simulink model "cm_sat_model"  (R2021b)
settings: Solver=ode23s  StartTime=0.0  StopTime=0.2  FixedStep=0.0001  MaxStep=1e-3  RelTol=5e-7  AbsTol=5e-7  EnableMultiTasking=on
values from neighbouring files (symbols this model uses):
  Dpsi = [ -2454.6 -2412.6 -2370.5 -2328.5 -2286.4 -2244.4 -2202.3  -2160.3 -2118.2 -2076.1 -2034.1 -1992.0 -1950.0 -1907.9 -1865.9  -1823.8 -1781.8 -1739.7 -1697.7 -1655.6 -1613.6 -1571.5 -1529.5  -1487.4 -1445.3 -1403.3 -1361.2 -1319.2 -1277.1 -1235.1 -1193.0  -1151.0 -1108.9 -1066.9 -1024.8 -982.76 -940.71 -898.65 -856.60  -814.55 -772.49 -730.44 -688.39 -646.43 -604.66 -562.89 -521.30  -479.53 -438.14  ...(+559 chars)    [cm_init.m]
  PAR = [wb r1 rp2 xl1 xlp2 xm]    [cm_init.m]
  psisat = [ -170.21 -169.93 -169.65 -169.36 -169.08 -168.80 -168.52  -168.23 -167.95 -167.67 -167.38 -167.10 -166.82 -166.54 -166.25  -165.97 -165.69 -165.40 -165.12 -164.84 -164.56 -164.27 -163.99  -163.71 -163.43 -163.14 -162.86 -162.58 -162.29 -162.01 -161.73  -161.45 -161.16 -160.88 -160.60 -160.32 -160.03 -159.75 -159.47  -159.18 -158.90 -158.62 -158.34 -157.96 -157.39 -156.83 -156.07  -155.51 -154.57  ...(+561 chars)    [cm_init.m]
  wb = 2*pi*F    (= 376.991118431)    [cm_init.m]
  XINIT = [0]    [cm_init.m]
undefined symbols (not defined in the file or in its folder): V1, V1f
settings Model: Creator=Alberto  LastModifiedBy=DELL
settings SolverCC: AutoScaleAbsTol=off  MaxOrder=4  AlgebraicLoopSolver=TrustRegion
settings DataIOCC: LimitDataPoints=on  SaveFormat=Array  SignalLoggingSaveFormat=ModelDataLogs  ReturnWorkspaceOutputs=off  SignalLoggingName=sigsOut
settings OptimizationCC: ExpressionDepthLimit=2147483647  LifeSpan=inf
settings DebuggingCC: AlgebraicLoopMsg=none  SaveWithParameterizedLinksMsg=none  UnderspecifiedInitializationDetection=Classic  MergeDetectMultiDrivingBlocksExec=none  SignalResolutionControl=TryResolveAllWithWarning  MultiTaskDSMMsg=warning  MultiTaskCondExecSysMsg=none  FcnCallInpInsideContextMsg=warning  StateNameClashWarn=warning  SFUnexpectedBacktrackingDiag=warning  SFNoUnconditionalDefaultTransitionDiag=warning  SFExecutionAtInitializationDiag=none  SFMachineParentedDataDiag=warning  ArithmeticOperatorsInVariantConditions=warning
settings HardwareCC: ProdBitPerPointer=32  ProdBitPerSizeT=32  ProdBitPerPtrDiffT=32  ProdLargestAtomicFloat=None  ProdIntDivRoundTo=Undefined  ProdEndianess=Unspecified  ProdWordSize=32  ProdHWDeviceType=32-bit Generic  TargetUnknown=on
settings ModelReferenceCC: PropagateSignalLabelsOutOfModel=off
settings SFSimCC: SimUseLocalCustomCode=off  CustomCodeUndefinedFunction=UseInterfaceOnly
settings RTWCC: RTWUseLocalCustomCode=off
settings CodeAppCC: StateflowObjectComments=on
settings GRTTargetCC: TargetLangStandard=C89/C90 (ANSI)  CombineOutputUpdateFcns=off  GRTInterface=on
settings ConfigComp: CovMetricSettings=dw  CovSaveCumulativeToWorkspaceVar=on  CovSaveSingleToWorkspaceVar=on  CovExternalEMLEnable=off

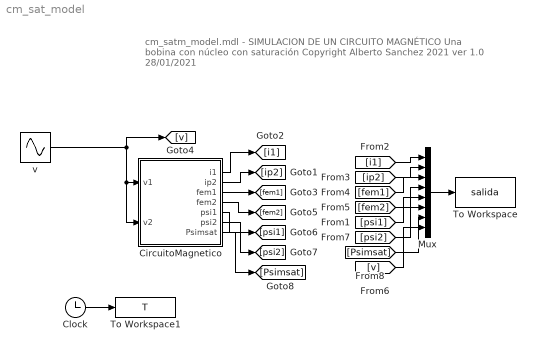
== system cm_sat_model ==
  note: cm_satm_model.mdl - SIMULACION DE UN CIRCUITO MAGNÉTICO
      | Una bobina con núcleo con saturación
      | Copyright Alberto Sanchez 2021
      | ver 1.0 28/01/2021
  CircuitoMagnetico : Subsystem
  Clock : Clock
  Mux : Mux  Inputs=8
  To Workspace : ToWorkspace  VariableName=salida  SampleTime=-1
  To Workspace1 : ToWorkspace  VariableName=T  SampleTime=-1
  v : Sin  Amplitude=V1  Frequency=wb  Phase=V1f  SampleTime=0
  wires:
  Clock/1 -> To Workspace1/1
  CircuitoMagnetico/2(ip2) -> [ip2]
  Mux/1 -> To Workspace/1
  CircuitoMagnetico/3(fem1) -> [fem1]
  CircuitoMagnetico/1(i1) -> [i1]
  CircuitoMagnetico/4(fem2) -> [fem2]
  v/1 -> CircuitoMagnetico/2(v2), CircuitoMagnetico/1(v1), [v]
  [i1] -> Mux/1
  [ip2] -> Mux/2
  [fem1] -> Mux/3
  [fem2] -> Mux/4
  CircuitoMagnetico/5(psi1) -> [psi1]
  CircuitoMagnetico/6(psi2) -> [psi2]
  CircuitoMagnetico/7(Psimsat) -> [Psimsat]
  [psi1] -> Mux/5
  [psi2] -> Mux/6
  [Psimsat] -> Mux/7
  [v] -> Mux/8

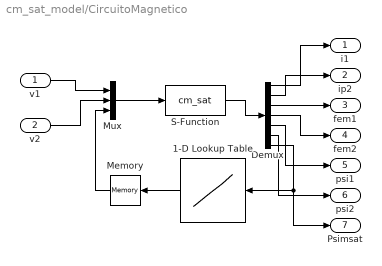
== system cm_sat_model/CircuitoMagnetico ==
  v1 : Inport
  v2 : Inport  Port=2
  1-D Lookup Table : Lookup_n-D  NumberOfTableDimensions=1  BreakpointsForDimension1=psisat  Table=Dpsi  RndMeth=Simplest  InputSameDT=on
  Demux : Demux  Outputs=7
      settings: DisplayOption=none
  Memory : Memory
  Mux : Mux  Inputs=3
  S-Function : S-Function  FunctionName=cm_sat  Parameters=XINIT,PAR  SFunctionDeploymentMode=off  EnableBusSupport=off
  i1 : Outport  VectorParamsAs1DForOutWhenUnconnected=off
  ip2 : Outport  Port=2  VectorParamsAs1DForOutWhenUnconnected=off
  fem1 : Outport  Port=3  VectorParamsAs1DForOutWhenUnconnected=off
  fem2 : Outport  Port=4  VectorParamsAs1DForOutWhenUnconnected=off
  psi1 : Outport  Port=5  VectorParamsAs1DForOutWhenUnconnected=off
  psi2 : Outport  Port=6  VectorParamsAs1DForOutWhenUnconnected=off
  Psimsat : Outport  Port=7  VectorParamsAs1DForOutWhenUnconnected=off
  wires:
  Mux/1 -> S-Function/1
  1-D Lookup Table/1 -> Memory/1
  S-Function/1 -> Demux/1
  v1/1 -> Mux/1
  v2/1 -> Mux/2
  Memory/1 -> Mux/3
  Demux/1 -> i1/1
  Demux/2 -> ip2/1
  Demux/3 -> fem1/1
  Demux/4 -> fem2/1
  Demux/5 -> psi1/1
  Demux/6 -> psi2/1
  Demux/7 -> 1-D Lookup Table/1, Psimsat/1
